simulink model "top_model"  (R2017b)
settings: Solver=FixedStepAuto  StartTime=0.0  StopTime=60000  FixedStep=.1  RelTol=1e-3  EnableMultiTasking=on
model workspace: external: MATLAB File C:\Users\Justin\Documents\00 MEng Project\PAN_ADCS\initialization\simulink_workspace_init.m (data not in the file)
undefined symbols (not defined in the file): h_init, hdmax, hmax, IAU, Imp_max, Imp_min, init, K_F, Kd, km, Kp, L_F, m_follower, match_tol, muE, ontime_max, ontime_min, q_init, s, Thrust_max, Thrust_min, wbn_init
libraries: aerolibtransform2 x9, hEemethod x8, aerolibconvert2 x6, aerolibgravity2 x5, sharedtransform x4, aerolibutil x4, aerolibcelestial x3, vrlib x2
(part 1 of 3)
settings Model: Creator=The MathWorks, Inc.  LastModifiedBy=Justin
settings DataIOCC: LimitDataPoints=on
settings OptimizationCC: LifeSpan=inf
settings DebuggingCC: AllowSymbolicDim=off  SFUnexpectedBacktrackingDiag=warning  SFNoUnconditionalDefaultTransitionDiag=warning  SFExecutionAtInitializationDiag=none
settings ModelReferenceCC: PropagateSignalLabelsOutOfModel=off
settings CodeAppCC: StateflowObjectComments=on
settings GRTTargetCC: TargetLangStandard=C89/C90 (ANSI)
settings ConfigComp: CovMetricSettings=dw  CovHtmlReporting=on  CovSaveCumulativeToWorkspaceVar=on  CovSaveSingleToWorkspaceVar=on  CovExternalEMLEnable=off

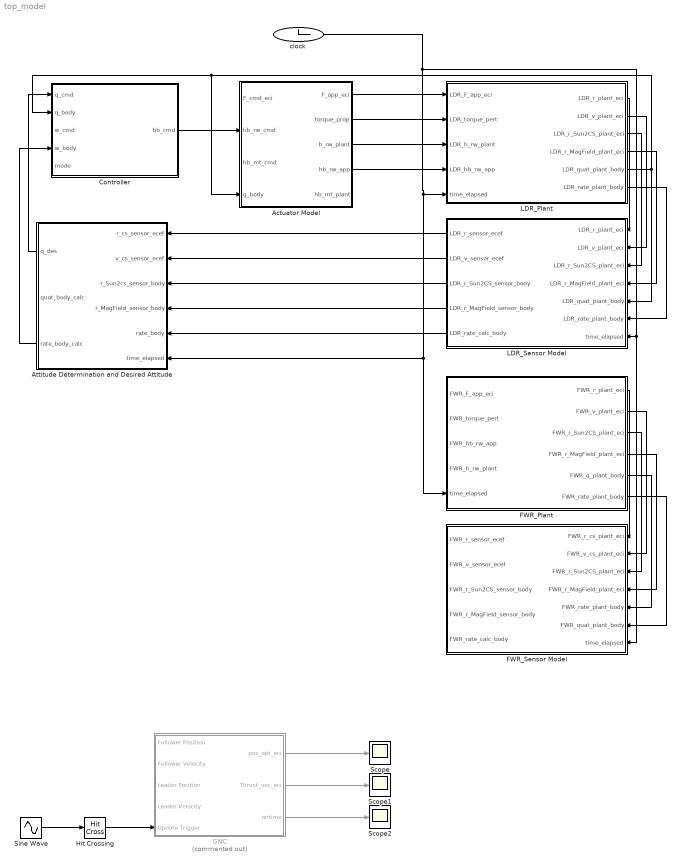
== system top_model ==
  Actuator Model : Subsystem
  Attitude Determination and Desired Attitude : Subsystem
  Controller : Subsystem
  FWR_Plant : Subsystem
  FWR_Sensor Model : Subsystem
  GNC : Subsystem  Commented=on
  Hit Crossing : HitCross  HitCrossingOffset=0.5  HitCrossingDirection=rising
  LDR_Plant : Subsystem
  LDR_Sensor Model : Subsystem
  Scope : Scope
  Scope1 : Scope
  Scope2 : Scope
  Sine Wave : Sin  Frequency=2*pi/5500  SampleTime=0
  clock : Clock
      settings: Decimation=100
  wires:
  clock/1 -> FWR_Sensor Model/7(time_elapsed), LDR_Sensor Model/7(time_elapsed), Attitude Determination and Desired Attitude/6(time_elapsed), FWR_Plant/5(time_elapsed), LDR_Plant/5(time_elapsed)
  LDR_Plant/1(LDR_r_plant_eci) -> LDR_Sensor Model/1(LDR_r_plant_eci)
  LDR_Plant/2(LDR_v_plant_eci) -> LDR_Sensor Model/2(LDR_v_plant_eci)
  LDR_Plant/3(LDR_r_Sun2CS_plant_eci) -> LDR_Sensor Model/3(LDR_r_Sun2CS_plant_eci)
  LDR_Plant/4(LDR_r_MagField_plant_eci) -> LDR_Sensor Model/4(LDR_r_MagField_plant_eci)
  LDR_Plant/6(LDR_rate_plant_body) -> LDR_Sensor Model/6(LDR_rate_plant_body)
  FWR_Plant/1(FWR_r_plant_eci) -> FWR_Sensor Model/1(FWR_r_cs_plant_eci)
  FWR_Plant/2(FWR_v_plant_eci) -> FWR_Sensor Model/2(FWR_v_cs_plant_eci)
  FWR_Plant/3(FWR_r_Sun2CS_plant_eci) -> FWR_Sensor Model/3(FWR_r_Sun2CS_plant_eci)
  FWR_Plant/4(FWR_r_MagField_plant_eci) -> FWR_Sensor Model/4(FWR_r_MagField_plant_eci)
  FWR_Plant/5(FWR_q_plant_body) -> FWR_Sensor Model/5(FWR_rate_plant_body)
  FWR_Plant/6(FWR_rate_plant_body) -> FWR_Sensor Model/6(FWR_quat_plant_body)
  Actuator Model/1(F_app_eci) -> LDR_Plant/1(LDR_F_app_eci)
  Actuator Model/2(torque_prop) -> LDR_Plant/2("LDR_torque_pert ")
  Actuator Model/3(h_rw_plant) -> LDR_Plant/3(LDR_h_rw_plant)
  Actuator Model/4(hb_rw_app) -> LDR_Plant/4(LDR_hb_rw_app)
  LDR_Sensor Model/1(LDR_r_sensor_ecef) -> Attitude Determination and Desired Attitude/1(r_cs_sensor_ecef)
  LDR_Sensor Model/2(LDR_v_sensor_ecef) -> Attitude Determination and Desired Attitude/2(v_cs_sensor_ecef)
  LDR_Sensor Model/3(LDR_r_Sun2CS_sensor_body) -> Attitude Determination and Desired Attitude/3(r_Sun2cs_sensor_body)
  LDR_Sensor Model/4(LDR_r_MagField_sensor_body) -> Attitude Determination and Desired Attitude/4(r_MagField_sensor_body)
  LDR_Sensor Model/5(LDR_rate_calc_body) -> Attitude Determination and Desired Attitude/5(rate_body)
  GNC/1(pos_opt_eci) -> Scope/1
  GNC/2(Thrust_vec_eci) -> Scope1/1
  GNC/3(ontime) -> Scope2/1
  Sine Wave/1 -> Hit Crossing/1
  Hit Crossing/1 -> GNC/5(Update Trigger)
  LDR_Plant/5(LDR_quat_plant_body) -> LDR_Sensor Model/5(LDR_quat_plant_body), Actuator Model/4(q_body), Controller/2(q_body)
  Attitude Determination and Desired Attitude/1(q_des) -> Controller/1(q_cmd)
  Attitude Determination and Desired Attitude/3(rate_body_calc) -> Controller/4(w_body)
  Controller/1(hb_cmd) -> Actuator Model/2(hb_rw_cmd)

== system top_model/Actuator Model ==
  F_cmd_eci : Inport
  hb_rw_cmd : Inport  Port=2
  hb_mt_cmd : Inport  Port=3
  q_body : Inport  Port=4
  Propulsion : Subsystem  Commented=on
  Rigid Body with Momentum Actuators and energy dissipation : Subsystem
  F_app_eci : Outport
  torque_prop : Outport  Port=2
  h_rw_plant : Outport  Port=3
  hb_rw_app : Outport  Port=4
  hb_mt_plant : Outport  Port=5
  wires:
  Rigid Body with Momentum Actuators and energy dissipation/1(LDR_h_RWA) -> h_rw_plant/1
  Rigid Body with Momentum Actuators and energy dissipation/2(LDR_hb_RWA) -> hb_rw_app/1
  hb_mt_cmd/1 -> hb_mt_plant/1
  F_cmd_eci/1 -> Propulsion/1(Force_cmd_eci)
  Propulsion/1(Force_applied) -> F_app_eci/1
  hb_rw_cmd/1 -> Rigid Body with Momentum Actuators and energy dissipation/1(hb)
  q_body/1 -> Rigid Body with Momentum Actuators and energy dissipation/2(q_body)

== system top_model/Attitude Determination and Desired Attitude ==
  r_cs_sensor_ecef : Inport
  v_cs_sensor_ecef : Inport  Port=2
  r_Sun2cs_sensor_body : Inport  Port=3
  r_MagField_sensor_body : Inport  Port=4
  rate_body : Inport  Port=5
  time_elapsed : Inport  Port=6
  Attitude Determination : Subsystem
  Demux1 : Demux
  Demux2 : Demux
  Direction Cosine Matrix to Quaternions : sharedtransform/Direction Cosine Matrix  to Quaternions  Commented=on
      settings: SourceProductName=Aerospace Blockset  SourceProductBaseCode=AE
  ECEF2ECI : Subsystem
  ECEF2ECI1 : Subsystem
  Position and Velocity to Desired Attitude in Quat : Subsystem
  Quaternions to Direction Cosine Matrix : sharedtransform/Quaternions to  Direction Cosine Matrix  Commented=on
      settings: SourceProductName=Aerospace Blockset  SourceProductBaseCode=AE
  Quaternions to Rotation Angles : sharedtransform/Quaternions to Rotation Angles  Commented=on  rotationOrder=ZYX
      settings: SourceProductBaseCode=AE
  Rotation Angles to Direction Cosine Matrix : sharedtransform/Rotation Angles to Direction Cosine Matrix  Commented=on  rotationOrder=ZYX
      settings: SourceProductBaseCode=AE
  q_calc : Scope  NumInputPorts=4
  q_ref : Scope  NumInputPorts=4
  q_des : Outport
  quat_body_calc : Outport  Port=2
  rate_body_calc : Outport  Port=3
  wires:
  rate_body/1 -> rate_body_calc/1
  time_elapsed/1 -> ECEF2ECI1/2(sec), ECEF2ECI/2(sec), Attitude Determination/1(time_elapsed)
  r_cs_sensor_ecef/1 -> ECEF2ECI/1(ecef)
  v_cs_sensor_ecef/1 -> ECEF2ECI1/1(ecef)
  ECEF2ECI/1(eci) -> Attitude Determination/2(r_cs_sensor_eci), Position and Velocity to Desired Attitude in Quat/1(r_cs_sensor_eci)
  ECEF2ECI1/1(eci) -> Position and Velocity to Desired Attitude in Quat/2(v_cs_sensor_eci)
  r_Sun2cs_sensor_body/1 -> Attitude Determination/3(r_Sun2cs_sensor_body)
  r_MagField_sensor_body/1 -> Attitude Determination/4(r_MagField_sensor_body)
  Attitude Determination/1(quat_body_calc) -> Demux1/1, quat_body_calc/1
  Demux1/2 -> q_calc/2
  Demux1/1 -> q_calc/1
  Demux1/3 -> q_calc/3
  Demux1/4 -> q_calc/4
  Position and Velocity to Desired Attitude in Quat/1(q_des) -> Demux2/1, q_des/1
  Demux2/2 -> q_ref/2
  Demux2/1 -> q_ref/1
  Demux2/3 -> q_ref/3
  Demux2/4 -> q_ref/4

== system top_model/Controller ==
  note: 0- Power ON / Restart
      | 1- Detumble
      | 2- Regulation Control
      | 3- Tracking Control
      | 4- Thermal Safe
      | 5- Power Max
      | 6- Large Angle Slew
  note: 0- Power ON/restart
      | 1- Safe hold
      | 2- Detumble
      | 3- Large angle slew
      | 4- Normal
      | 5- Eclipse
      | 6- Docking
  q_cmd : Inport
  q_body : Inport  Port=2
  w_cmd : Inport  Port=3
  w_body : Inport  Port=4
  mode : Inport  Port=5
  Free Rigid Body with Momentum Actuators2 : Subsystem  Commented=on
  If : If  IfExpression=u1 == 0  ElseIfExpressions=u1 == 1, u1 == 2, u1 == 3, u1 == 4, u1==5
  Mode Generator : Stateflow chart  Commented=on  TreatAsAtomicUnit=on
  Normal Mode Control System : Subsystem  TreatAsAtomicUnit=on
  TestNormalMode : Constant  Value=4
  hb_cmd : Outport
  wires:
  q_cmd/1 -> Mode Generator/2(q_cmd), Normal Mode Control System/1(q_cmd)
  q_body/1 -> Mode Generator/1(q_body), Normal Mode Control System/2(q_body)
  w_cmd/1 -> Normal Mode Control System/3(w_cmd)
  w_body/1 -> Mode Generator/3(w_body), Normal Mode Control System/4(w_body)
  TestNormalMode/1 -> If/1
  If/5 -> Normal Mode Control System/Action
  Normal Mode Control System/1(hb_cmd) -> hb_cmd/1

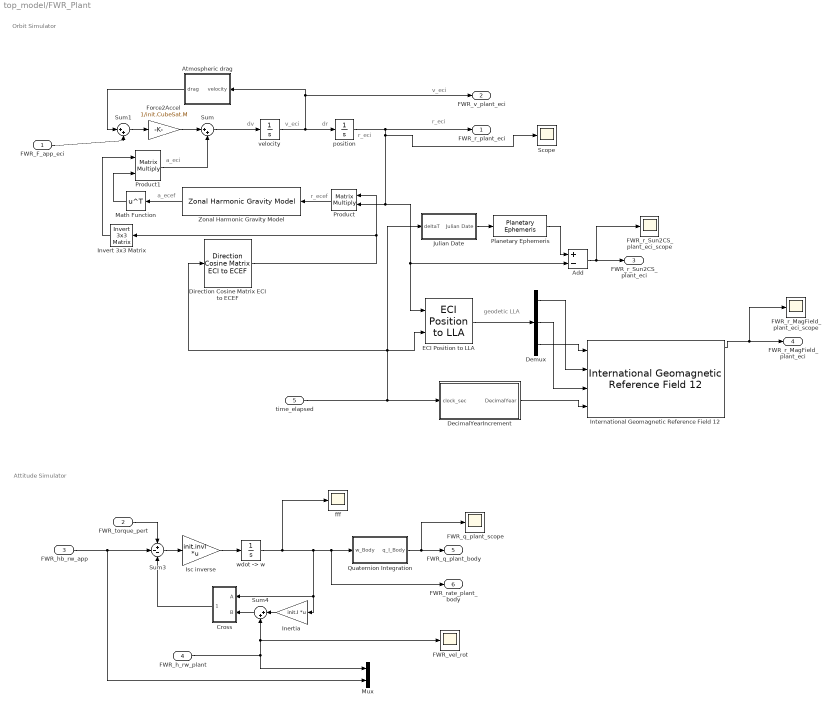
== system top_model/FWR_Plant ==
  note: Attitude Simulator
  note: dr
  note: r_eci
  note: r_eci
  note: dv
  note: v_eci
  note: Orbit Simulator
  note: r_ecef
  note: geodetic LLA
  note: a_eci
  note: v_eci
  note: a_ecef
  FWR_F_app_eci : Inport
  "FWR_torque_pert " : Inport  Port=2
  FWR_hb_rw_app : Inport  Port=3
  FWR_h_rw_plant : Inport  Port=4
  time_elapsed : Inport  Port=5
  Add : Sum  Inputs=+-
  Atmospheric drag : MATLAB Function  TreatAsAtomicUnit=on
  Cross : Subsystem
  DecimalYearIncrement : Subsystem
  Demux : Demux  Outputs=3
  Direction Cosine Matrix ECI to ECEF : aerolibtransform2/Direction Cosine Matrix ECI to ECEF  red=IAU-2000/2006  year=init.year  month=October  day=20  hour=init.hour  min=init.min  sec=init.sec  deltaT=Sec  errorflag=Error  extraparamflag=off
      settings: AttributesFormatString=%<red>  SourceProductName=Aerospace Blockset  SourceProductBaseCode=AE
  ECI Position to LLA : aerolibtransform2/ECI Position to LLA  red=IAU-2000/2006  year=init.year  month=October  day=20  hour=init.hour  min=init.min  sec=init.sec  deltaT=Sec  errorflag=Error  extraparamflag=off  eunits=Metric (MKS)  earthmodel=WGS84  flat=1/298.257223563  eqradius=6378137
      settings: AttributesFormatString=%<red>  SourceProductName=Aerospace Blockset  SourceProductBaseCode=AE
  FWR_q_plant_scope : Scope
  FWR_r_MagField_plant_eci_scope : Scope
  FWR_r_Sun2CS_plant_eci_scope : Scope
  "FWR_vel_rot " : Scope
  Force2Accel : Gain  Gain=1/init.CubeSat.M
  Inertia : Gain  Gain=init.I  Multiplication=Matrix(K*u)  SaturateOnIntegerOverflow=on  OutDataTypeStr=Inherit: Same as input  ParamDataTypeStr=Inherit: Same as input
  International Geomagnetic Reference Field 12 : aerolibgravity2/International Geomagnetic Reference Field 12  units=Metric (MKS)  time_in=on  month=January  day=1  year=2020  action=None  sv_out=off
      settings: SourceProductName=Aerospace Blockset  SourceProductBaseCode=AE
  Invert 3x3 Matrix : aerolibutil/Invert  3x3 Matrix
  Isc inverse : Gain  Gain=init.invI  Multiplication=Matrix(K*u)  SaturateOnIntegerOverflow=on  OutDataTypeStr=Inherit: Same as input  ParamDataTypeStr=Inherit: Same as input
  Julian Date : Subsystem
  Math Function : Math  Operator=transpose  SaturateOnIntegerOverflow=on
  Mux : Mux  Inputs=2
  Planetary Ephemeris : aerolibcelestial/Planetary Ephemeris  kmflag=km,km/s  epochflag=Julian date  de=DE430  nCenter=Earth  nTarget=Sun  errorflag=Error  velflag=off
      settings: SourceProductName=Aerospace Blockset  SourceProductBaseCode=AE
  Product : Product  Multiplication=Matrix(*)
  Product1 : Product  Multiplication=Matrix(*)
  Quaternion Integration : Subsystem
  Scope : Scope
  Sum : Sum  Inputs=|++
  Sum1 : Sum  Inputs=|++
  Sum3 : Sum  Inputs=+--  SaturateOnIntegerOverflow=on  InputSameDT=on  OutDataTypeStr=Inherit: Same as first input
  Sum4 : Sum  Inputs=|++
  Zonal Harmonic Gravity Model : aerolibgravity2/Zonal Harmonic Gravity Model  units=Metric (MKS)  degree=4  action=Warning  ptype=Earth  R=6378136.3  GM=398600441500000  jvalue=[1.0826269e-03 -2.5323000e-06 -1.6204000e-06]
      settings: SourceProductName=Aerospace Blockset  SourceProductBaseCode=AE
  fff : Scope
  position : Integrator  InitialCondition=init.FWR.P  ContinuousStateAttributes='position'
  velocity : Integrator  InitialCondition=init.FWR.V  ContinuousStateAttributes='velocity'
  "wdot -> w" : Integrator  InitialCondition=init.FWR.wbn
  FWR_r_plant_eci : Outport
  FWR_v_plant_eci : Outport  Port=2
  FWR_r_Sun2CS_plant_eci : Outport  Port=3
  FWR_r_MagField_plant_eci : Outport  Port=4
  FWR_q_plant_body : Outport  Port=5
  FWR_rate_plant_body : Outport  Port=6
  wires:
  Inertia/1 -> Sum4/1
  Quaternion Integration/1(q_I_Body) -> FWR_q_plant_scope/1, FWR_q_plant_body/1
  FWR_hb_rw_app/1 -> Sum3/2, Mux/2
  Sum3/1 -> Isc inverse/1
  "wdot -> w"/1 -> Quaternion Integration/1(w_Body), FWR_rate_plant_body/1, Cross/1(A), Inertia/1, fff/1
  Isc inverse/1 -> "wdot -> w"/1
  "FWR_torque_pert "/1 -> Sum3/1
  Sum4/1 -> Cross/2(B)
  Cross/1(AxB) -> Sum3/3
  FWR_h_rw_plant/1 -> Sum4/2, "FWR_vel_rot "/1, Mux/1
  time_elapsed/1 -> DecimalYearIncrement/1(clock_sec), ECI Position to LLA/2, Direction Cosine Matrix ECI to ECEF/1, Julian Date/1(deltaT)
  DecimalYearIncrement/1(DecimalYear) -> International Geomagnetic Reference Field 12/4
  International Geomagnetic Reference Field 12/1 -> FWR_r_MagField_plant_eci_scope/1, FWR_r_MagField_plant_eci/1
  Planetary Ephemeris/1 -> Add/1
  velocity/1 -> position/1, Atmospheric drag/1(velocity), FWR_v_plant_eci/1
  Force2Accel/1 -> Sum/1
  Demux/3 -> International Geomagnetic Reference Field 12/1
  Math Function/1 -> Product1/2
  Sum/1 -> velocity/1
  Product1/1 -> Sum/2
  Demux/1 -> International Geomagnetic Reference Field 12/2
  Atmospheric drag/1(drag) -> Sum1/1
  Product/1 -> Zonal Harmonic Gravity Model/1
  FWR_F_app_eci/1 -> Sum1/2
  Zonal Harmonic Gravity Model/1 -> Math Function/1
  position/1 -> Product/2, ECI Position to LLA/1, Add/2, Scope/1, FWR_r_plant_eci/1
  Demux/2 -> International Geomagnetic Reference Field 12/3
  Direction Cosine Matrix ECI to ECEF/1 -> Invert 3x3 Matrix/1, Product/1
  Invert 3x3 Matrix/1 -> Product1/1
  Julian Date/1(Julian Date) -> Planetary Ephemeris/1
  Sum1/1 -> Force2Accel/1
  ECI Position to LLA/1 -> Demux/1
  Add/1 -> FWR_r_Sun2CS_plant_eci_scope/1, FWR_r_Sun2CS_plant_eci/1

== system top_model/FWR_Sensor Model ==
  note: Gyroscope
  note: Magnetometer
  note: Sun Sensor
  note: GPS
  note: GPS
  FWR_r_cs_plant_eci : Inport
  FWR_v_cs_plant_eci : Inport  Port=2
  FWR_r_Sun2CS_plant_eci : Inport  Port=3
  FWR_r_MagField_plant_eci : Inport  Port=4
  FWR_rate_plant_body : Inport  Port=5
  FWR_quat_plant_body : Inport  Port=6
  time_elapsed : Inport  Port=7
  Direction Cosine Matrix ECI to ECEF : aerolibtransform2/Direction Cosine Matrix ECI to ECEF  red=IAU-2000/2006  year=init.year  month=October  day=20  hour=init.hour  min=init.min  sec=init.sec  deltaT=Sec  errorflag=Error  extraparamflag=off
      settings: AttributesFormatString=%<red>  SourceProductName=Aerospace Blockset  SourceProductBaseCode=AE
  Matrix Multiply : Product  Multiplication=Matrix(*)
  Matrix Multiply1 : Product  Multiplication=Matrix(*)
  FWR_r_sensor_ecef : Outport
  FWR_v_sensor_ecef : Outport  Port=2
  FWR_r_Sun2CS_sensor_body : Outport  Port=3
  FWR_r_MagField_sensor_body : Outport  Port=4
  FWR_rate_calc_body : Outport  Port=5
  wires:
  FWR_r_cs_plant_eci/1 -> Matrix Multiply/2
  FWR_r_Sun2CS_plant_eci/1 -> FWR_r_Sun2CS_sensor_body/1
  FWR_r_MagField_plant_eci/1 -> FWR_r_MagField_sensor_body/1
  FWR_rate_plant_body/1 -> FWR_rate_calc_body/1
  FWR_quat_plant_body/1 -> ?
  time_elapsed/1 -> Direction Cosine Matrix ECI to ECEF/1
  Direction Cosine Matrix ECI to ECEF/1 -> Matrix Multiply1/1, Matrix Multiply/1
  Matrix Multiply/1 -> FWR_r_sensor_ecef/1
  FWR_v_cs_plant_eci/1 -> Matrix Multiply1/2
  Matrix Multiply1/1 -> FWR_v_sensor_ecef/1

== system top_model/GNC ==
  Follower Position : Inport
  Follower Velocity : Inport  Port=2
  Leader Position : Inport  Port=3
  Leader Velocity : Inport  Port=4
  Update Trigger : Inport  Port=5
  Follower Maneuver : Subsystem
  Follower Orbital Elements : Subsystem
  Leader Orbital Elements : Subsystem
  Mux : Mux  Inputs=6
  Mux1 : Mux  Inputs=6
  Params : Subsystem
  Target Orbit : MATLAB Function  TreatAsAtomicUnit=on
  pos_opt_eci : Outport
  Thrust_vec_eci : Outport  Port=2
  ontime : Outport  Port=3
  wires:
  Follower Position/1 -> Follower Orbital Elements/1(r), Follower Maneuver/1(r_follower), Target Orbit/3(r_f)
  Follower Maneuver/2(pos_opt) -> pos_opt_eci/1
  [Imp_min] -> Follower Maneuver/7(Imp_min)
  Follower Maneuver/3(Thrust_vec) -> Thrust_vec_eci/1
  Leader Orbital Elements/4(Ω) -> Mux/4
  Mux/1 -> Target Orbit/5(els_t)
  Follower Orbital Elements/6(θ) -> Mux1/6
  Follower Orbital Elements/2(e) -> Mux1/2
  Follower Orbital Elements/3(i) -> Mux1/3
  Update Trigger/1 -> Follower Maneuver/8(Update Trigger)
  Leader Velocity/1 -> Leader Orbital Elements/2(v), Target Orbit/2(v_t)
  [Imp_max] -> Follower Maneuver/6(Imp_max)
  Target Orbit/1(x_tgt) -> Follower Maneuver/4(x_tgt)
  [muE] -> Follower Maneuver/3(mu), Target Orbit/7(muE)
  [match_tol] -> Target Orbit/9(match_tol)
  [m_f] -> Follower Maneuver/5(m_follower)
  Follower Velocity/1 -> Follower Orbital Elements/2(v), Follower Maneuver/2(v_follower), Target Orbit/4(v_f)
  Follower Orbital Elements/1(a) -> Mux1/1
  Follower Orbital Elements/4(Ω) -> Mux1/4
  Leader Orbital Elements/5(ω) -> Mux/5
  Follower Maneuver/4(ontime) -> ontime/1
  Mux1/1 -> Target Orbit/6(els_f)
  Leader Orbital Elements/3(i) -> Mux/3
  Follower Orbital Elements/5(ω) -> Mux1/5
  Leader Orbital Elements/6(θ) -> Mux/6
  Leader Position/1 -> Leader Orbital Elements/1(r), Target Orbit/1(r_t)
  Leader Orbital Elements/1(a) -> Mux/1
  Leader Orbital Elements/2(e) -> Mux/2
  [K_F] -> Target Orbit/8(K_F)

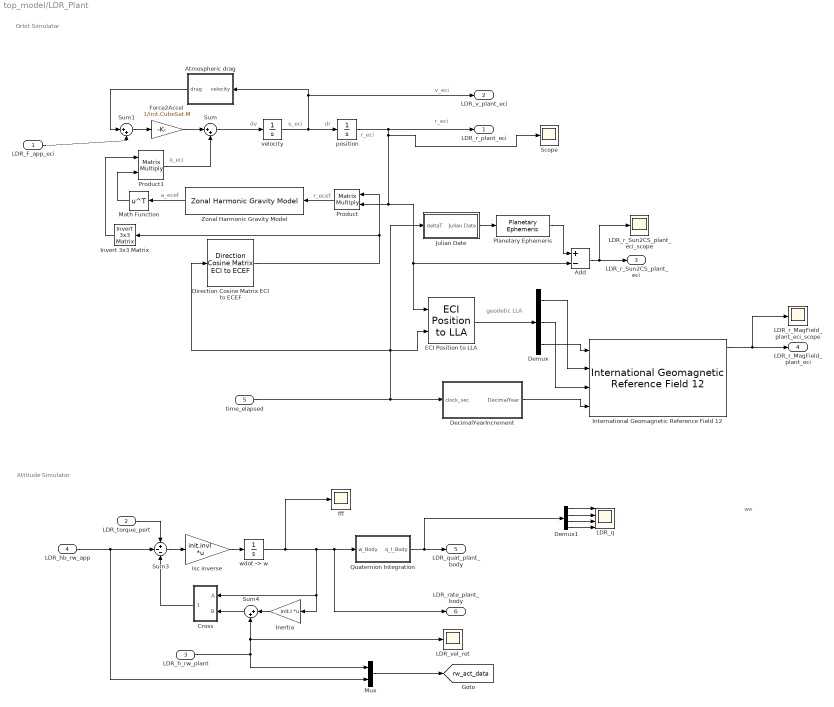
== system top_model/LDR_Plant ==
  note: we
  note: a_ecef
  note: v_eci
  note: a_eci
  note: geodetic LLA
  note: r_ecef
  note: Orbit Simulator
  note: v_eci
  note: dv
  note: r_eci
  note: r_eci
  note: dr
  note: Attitude Simulator
  LDR_F_app_eci : Inport
  "LDR_torque_pert " : Inport  Port=2
  LDR_h_rw_plant : Inport  Port=3
  LDR_hb_rw_app : Inport  Port=4
  time_elapsed : Inport  Port=5
  Add : Sum  Inputs=+-
  Atmospheric drag : MATLAB Function  TreatAsAtomicUnit=on
  Cross : Subsystem
  DecimalYearIncrement : Subsystem
  Demux : Demux  Outputs=3
  Demux1 : Demux
  Direction Cosine Matrix ECI to ECEF : aerolibtransform2/Direction Cosine Matrix ECI to ECEF  red=IAU-2000/2006  year=init.year  month=October  day=20  hour=init.hour  min=init.min  sec=init.sec  deltaT=Sec  errorflag=Error  extraparamflag=off
      settings: AttributesFormatString=%<red>  SourceProductName=Aerospace Blockset  SourceProductBaseCode=AE
  ECI Position to LLA : aerolibtransform2/ECI Position to LLA  red=IAU-2000/2006  year=init.year  month=October  day=20  hour=init.hour  min=init.min  sec=init.sec  deltaT=Sec  errorflag=Error  extraparamflag=off  eunits=Metric (MKS)  earthmodel=WGS84  flat=1/298.257223563  eqradius=6378137
      settings: AttributesFormatString=%<red>  SourceProductName=Aerospace Blockset  SourceProductBaseCode=AE
  Force2Accel : Gain  Gain=1/init.CubeSat.M
  Inertia : Gain  Gain=init.I  Multiplication=Matrix(K*u)  SaturateOnIntegerOverflow=on  OutDataTypeStr=Inherit: Same as input  ParamDataTypeStr=Inherit: Same as input
  International Geomagnetic Reference Field 12 : aerolibgravity2/International Geomagnetic Reference Field 12  units=Metric (MKS)  time_in=on  month=January  day=1  year=2020  action=None  sv_out=off
      settings: SourceProductName=Aerospace Blockset  SourceProductBaseCode=AE
  Invert 3x3 Matrix : aerolibutil/Invert  3x3 Matrix
  Isc inverse : Gain  Gain=init.invI  Multiplication=Matrix(K*u)  SaturateOnIntegerOverflow=on  OutDataTypeStr=Inherit: Same as input  ParamDataTypeStr=Inherit: Same as input
  Julian Date : Subsystem
  LDR_q : Scope  NumInputPorts=4
  LDR_r_MagField_plant_eci_scope : Scope
  LDR_r_Sun2CS_plant_eci_scope : Scope
  "LDR_vel_rot " : Scope
  Math Function : Math  Operator=transpose  SaturateOnIntegerOverflow=on
  Mux : Mux  Inputs=2
  Planetary Ephemeris : aerolibcelestial/Planetary Ephemeris  kmflag=km,km/s  epochflag=Julian date  de=DE430  nCenter=Earth  nTarget=Sun  errorflag=Error  velflag=off
      settings: SourceProductName=Aerospace Blockset  SourceProductBaseCode=AE
  Product : Product  Multiplication=Matrix(*)
  Product1 : Product  Multiplication=Matrix(*)
  Quaternion Integration : Subsystem
  Scope : Scope
  Sum : Sum  Inputs=|++
  Sum1 : Sum  Inputs=|++
  Sum3 : Sum  Inputs=+--  SaturateOnIntegerOverflow=on  InputSameDT=on  OutDataTypeStr=Inherit: Same as first input
  Sum4 : Sum  Inputs=|++
  Zonal Harmonic Gravity Model : aerolibgravity2/Zonal Harmonic Gravity Model  units=Metric (MKS)  degree=4  action=Warning  ptype=Earth  R=6378136.3  GM=398600441500000  jvalue=[1.0826269e-03 -2.5323000e-06 -1.6204000e-06]
      settings: SourceProductName=Aerospace Blockset  SourceProductBaseCode=AE
  fff : Scope
  position : Integrator  InitialCondition=init.LDR.P  ContinuousStateAttributes='position'
  velocity : Integrator  InitialCondition=init.LDR.V  ContinuousStateAttributes='velocity'
  "wdot -> w" : Integrator  InitialCondition=init.LDR.wbn
  LDR_r_plant_eci : Outport
  LDR_v_plant_eci : Outport  Port=2
  LDR_r_Sun2CS_plant_eci : Outport  Port=3
  LDR_r_MagField_plant_eci : Outport  Port=4
  LDR_quat_plant_body : Outport  Port=5
  LDR_rate_plant_body : Outport  Port=6
  tag scope: rw_act_data=global
  wires:
  Add/1 -> LDR_r_Sun2CS_plant_eci/1, LDR_r_Sun2CS_plant_eci_scope/1
  ECI Position to LLA/1 -> Demux/1
  Sum1/1 -> Force2Accel/1
  Julian Date/1(Julian Date) -> Planetary Ephemeris/1
  Invert 3x3 Matrix/1 -> Product1/1
  Direction Cosine Matrix ECI to ECEF/1 -> Product/1, Invert 3x3 Matrix/1
  Demux/2 -> International Geomagnetic Reference Field 12/3
  Zonal Harmonic Gravity Model/1 -> Math Function/1
  LDR_F_app_eci/1 -> Sum1/2
  Product/1 -> Zonal Harmonic Gravity Model/1
  Atmospheric drag/1(drag) -> Sum1/1
  Demux/1 -> International Geomagnetic Reference Field 12/2
  Product1/1 -> Sum/2
  Sum/1 -> velocity/1
  Math Function/1 -> Product1/2
  Demux/3 -> International Geomagnetic Reference Field 12/1
  Force2Accel/1 -> Sum/1
  velocity/1 -> LDR_v_plant_eci/1, Atmospheric drag/1(velocity), position/1
  Planetary Ephemeris/1 -> Add/1
  International Geomagnetic Reference Field 12/1 -> LDR_r_MagField_plant_eci/1, LDR_r_MagField_plant_eci_scope/1
  DecimalYearIncrement/1(DecimalYear) -> International Geomagnetic Reference Field 12/4
  time_elapsed/1 -> Julian Date/1(deltaT), Direction Cosine Matrix ECI to ECEF/1, ECI Position to LLA/2, DecimalYearIncrement/1(clock_sec)
  LDR_h_rw_plant/1 -> Mux/1, "LDR_vel_rot "/1, Sum4/2
  Cross/1(AxB) -> Sum3/3
  Sum4/1 -> Cross/2(B)
  "LDR_torque_pert "/1 -> Sum3/1
  Isc inverse/1 -> "wdot -> w"/1
  "wdot -> w"/1 -> fff/1, Inertia/1, Cross/1(A), LDR_rate_plant_body/1, Quaternion Integration/1(w_Body)
  Sum3/1 -> Isc inverse/1
  LDR_hb_rw_app/1 -> Mux/2, Sum3/2
  Mux/1 -> [rw_act_data]
  Inertia/1 -> Sum4/1
  Quaternion Integration/1(q_I_Body) -> Demux1/1, LDR_quat_plant_body/1
  Demux1/2 -> LDR_q/2
  Demux1/1 -> LDR_q/1
  Demux1/3 -> LDR_q/3
  Demux1/4 -> LDR_q/4
  position/1 -> LDR_r_plant_eci/1, Scope/1, Add/2, ECI Position to LLA/1, Product/2

== system top_model/LDR_Sensor Model ==
  note: Gyroscope
  note: Magnetometer
  note: Sun Sensor
  note: GPS
  note: GPS
  LDR_r_plant_eci : Inport
  LDR_v_plant_eci : Inport  Port=2
  LDR_r_Sun2CS_plant_eci : Inport  Port=3
  LDR_r_MagField_plant_eci : Inport  Port=4
  LDR_quat_plant_body : Inport  Port=5
  LDR_rate_plant_body : Inport  Port=6
  time_elapsed : Inport  Port=7
  Direction Cosine Matrix ECI to ECEF : aerolibtransform2/Direction Cosine Matrix ECI to ECEF  red=IAU-2000/2006  year=init.year  month=October  day=20  hour=init.hour  min=init.min  sec=init.sec  deltaT=Sec  errorflag=Error  extraparamflag=off
      settings: AttributesFormatString=%<red>  SourceProductName=Aerospace Blockset  SourceProductBaseCode=AE
  Matrix Multiply{,1..3} (4 alike) : Product  Multiplication=Matrix(*)
  quat to DCM : Subsystem  mask(Direction Cosine Matrix){}
      mask help: Determines the 3x3 Direction Cosine Matrix (DCM) from a 4x1 quaternion orientation vector. The outputted DCM transforms vectors from inertial axes to body axes. This version corrects the fucked-up MATLAB one.
      mask Help:
      | <p>This block determines the 3x3 Direction Cosine Matrix (DCM) from a 4x1 quaternion orientation vector. The outputted DCM transforms vectors from inertial axes to body axes.  This version corrects the fucked-up MATLAB one</p>
      | 
      | <p>The block input and output contain more than one signal as described below.</p>
      | 
      | <p><H4>Block Vector Input - Quaternion</H4>
      | <ul>
      | <li>q0</li>
      | <li>q1</li>
      | <li>q2</li>
      | <li>q3</li>
      | </ul>
      | </p>
      | 
      | <p><H4>Block Matrix Output - Direction Cosine Matrix  </H4>
      |     <ul>
      |    </ul>
      |    </p>
      mask Display: disp('q to Q')
  LDR_r_sensor_ecef : Outport
  LDR_v_sensor_ecef : Outport  Port=2
  LDR_r_Sun2CS_sensor_body : Outport  Port=3
  LDR_r_MagField_sensor_body : Outport  Port=4
  LDR_rate_calc_body : Outport  Port=5
  wires:
  LDR_r_plant_eci/1 -> Matrix Multiply/2
  LDR_rate_plant_body/1 -> LDR_rate_calc_body/1
  LDR_quat_plant_body/1 -> quat to DCM/1(e0 e1 e2 e3)
  time_elapsed/1 -> Direction Cosine Matrix ECI to ECEF/1
  Direction Cosine Matrix ECI to ECEF/1 -> Matrix Multiply1/1, Matrix Multiply/1
  Matrix Multiply/1 -> LDR_r_sensor_ecef/1
  LDR_v_plant_eci/1 -> Matrix Multiply1/2
  Matrix Multiply1/1 -> LDR_v_sensor_ecef/1
  LDR_r_Sun2CS_plant_eci/1 -> Matrix Multiply3/2
  LDR_r_MagField_plant_eci/1 -> Matrix Multiply2/2
  Matrix Multiply3/1 -> LDR_r_Sun2CS_sensor_body/1
  Matrix Multiply2/1 -> LDR_r_MagField_sensor_body/1
  quat to DCM/1(DCM) -> Matrix Multiply3/1, Matrix Multiply2/1

== system top_model/Actuator Model/Propulsion ==
  Force_cmd_eci : Inport
  MATLAB Function : MATLAB Function  TreatAsAtomicUnit=on
  Force_applied : Outport
  wires:
  Force_cmd_eci/1 -> MATLAB Function/1(Target)

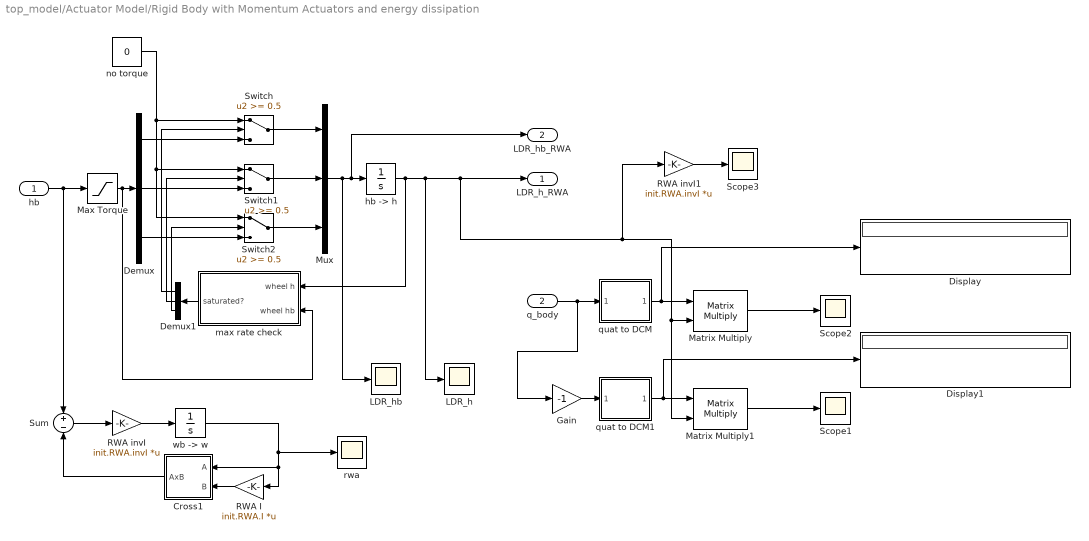
== system top_model/Actuator Model/Rigid Body with Momentum Actuators and energy dissipation ==
  hb : Inport
  q_body : Inport  Port=2
  Cross1 : Subsystem
  Demux : Demux  Outputs=3
  Demux1 : Demux  Outputs=3
  Display : Display
  Display1 : Display
  Gain : Gain  Gain=-1
  LDR_h : Scope
  LDR_hb : Scope
  Matrix Multiply : Product  Multiplication=Matrix(*)
  Matrix Multiply1 : Product  Multiplication=Matrix(*)
  Max Torque : Saturate  UpperLimit=init.hdmax  LowerLimit=-init.hdmax
  Mux : Mux  Inputs=3
  RWA I : Gain  Gain=init.RWA.I  Multiplication=Matrix(K*u)
  RWA invI : Gain  Gain=init.RWA.invI  Multiplication=Matrix(K*u)
  RWA invI1 : Gain  Gain=init.RWA.invI  Multiplication=Matrix(K*u)
  Scope1 : Scope
  Scope2 : Scope
  Scope3 : Scope
  Sum : Sum  Inputs=+|-
  Switch : Switch  Threshold=0.5  SaturateOnIntegerOverflow=on  InputSameDT=on
  Switch1 : Switch  Threshold=0.5  SaturateOnIntegerOverflow=on  InputSameDT=on
  Switch2 : Switch  Threshold=0.5  SaturateOnIntegerOverflow=on  InputSameDT=on
  "hb -> h" : Integrator  InitialCondition=init.LDR.h
  max rate check : Subsystem
  no torque : Constant  Value=0
  quat to DCM : Subsystem  mask(Direction Cosine Matrix){}
      mask help: Determines the 3x3 Direction Cosine Matrix (DCM) from a 4x1 quaternion orientation vector. The outputted DCM transforms vectors from inertial axes to body axes. This version corrects the fucked-up MATLAB one.
      mask Help:
      | <p>This block determines the 3x3 Direction Cosine Matrix (DCM) from a 4x1 quaternion orientation vector. The outputted DCM transforms vectors from inertial axes to body axes.  This version corrects the fucked-up MATLAB one</p>
      | 
      | <p>The block input and output contain more than one signal as described below.</p>
      | 
      | <p><H4>Block Vector Input - Quaternion</H4>
      | <ul>
      | <li>q0</li>
      | <li>q1</li>
      | <li>q2</li>
      | <li>q3</li>
      | </ul>
      | </p>
      | 
      | <p><H4>Block Matrix Output - Direction Cosine Matrix  </H4>
      |     <ul>
      |    </ul>
      |    </p>
      mask Display: disp('q to Q')
  quat to DCM1 : Subsystem  mask(Direction Cosine Matrix){}
      mask help: Determines the 3x3 Direction Cosine Matrix (DCM) from a 4x1 quaternion orientation vector. The outputted DCM transforms vectors from inertial axes to body axes. This version corrects the fucked-up MATLAB one.
      mask Help:
      | <p>This block determines the 3x3 Direction Cosine Matrix (DCM) from a 4x1 quaternion orientation vector. The outputted DCM transforms vectors from inertial axes to body axes.  This version corrects the fucked-up MATLAB one</p>
      | 
      | <p>The block input and output contain more than one signal as described below.</p>
      | 
      | <p><H4>Block Vector Input - Quaternion</H4>
      | <ul>
      | <li>q0</li>
      | <li>q1</li>
      | <li>q2</li>
      | <li>q3</li>
      | </ul>
      | </p>
      | 
      | <p><H4>Block Matrix Output - Direction Cosine Matrix  </H4>
      |     <ul>
      |    </ul>
      |    </p>
      mask Display: disp('q to Q')
  rwa : Scope
  "wb -> w" : Integrator  InitialCondition=[0;0;0]
  LDR_h_RWA : Outport
  LDR_hb_RWA : Outport  Port=2
  wires:
  hb/1 -> Max Torque/1, Sum/1
  Mux/1 -> LDR_hb_RWA/1, "hb -> h"/1, LDR_hb/1
  Max Torque/1 -> Demux/1, max rate check/2(wheel hb)
  max rate check/1(saturated?) -> Demux1/1
  Demux1/1 -> Switch/2
  Demux1/2 -> Switch1/2
  Demux1/3 -> Switch2/2
  no torque/1 -> Switch/1, Switch1/1, Switch2/1
  Demux/1 -> Switch/3
  Demux/2 -> Switch1/3
  Demux/3 -> Switch2/3
  Switch/1 -> Mux/1
  Switch1/1 -> Mux/2
  Switch2/1 -> Mux/3
  q_body/1 -> Gain/1, quat to DCM/1(e0 e1 e2 e3)
  quat to DCM/1(DCM) -> Display/1, Matrix Multiply/1
  Matrix Multiply/1 -> Scope2/1
  Matrix Multiply1/1 -> Scope1/1
  quat to DCM1/1(DCM) -> Display1/1, Matrix Multiply1/1
  "hb -> h"/1 -> max rate check/1(wheel h), RWA invI1/1, Matrix Multiply1/2, Matrix Multiply/2, LDR_h_RWA/1, LDR_h/1
  Gain/1 -> quat to DCM1/1(e0 e1 e2 e3)
  RWA I/1 -> Cross1/2(B)
  "wb -> w"/1 -> rwa/1, Cross1/1(A), RWA I/1
  Cross1/1(AxB) -> Sum/2
  Sum/1 -> RWA invI/1
  RWA invI/1 -> "wb -> w"/1
  RWA invI1/1 -> Scope3/1

== system top_model/Attitude Determination and Desired Attitude/Attitude Determination ==
  time_elapsed : Inport
  r_cs_sensor_eci : Inport  Port=2
  r_Sun2cs_sensor_body : Inport  Port=3
  r_MagField_sensor_body : Inport  Port=4
  Generate reference vectors from Ephemeris and Magnetic Field Model : Subsystem
  Subsystem : Subsystem
  quat_body_calc : Outport
  wires:
  r_cs_sensor_eci/1 -> Generate reference vectors from Ephemeris and Magnetic Field Model/2(r_cs_sensor_eci)
  time_elapsed/1 -> Generate reference vectors from Ephemeris and Magnetic Field Model/1(time_elapsed)
  r_Sun2cs_sensor_body/1 -> Subsystem/3(r_Sun2cs_sensor_body)
  r_MagField_sensor_body/1 -> Subsystem/4(r_MagField_sensor_body)
  Generate reference vectors from Ephemeris and Magnetic Field Model/1(r_Sun2cs_ref_eci) -> Subsystem/1(r_Sun2cs_ref_eci)
  Generate reference vectors from Ephemeris and Magnetic Field Model/2(r_MagField_ref_eci) -> Subsystem/2(r_MagField_ref_eci)
  Subsystem/1(quat_body_calc) -> quat_body_calc/1

== system top_model/Attitude Determination and Desired Attitude/ECEF2ECI ==
  ecef : Inport
  sec : Inport  Port=2
  Direction Cosine Matrix ECI to ECEF : aerolibtransform2/Direction Cosine Matrix ECI to ECEF  red=IAU-2000/2006  year=init.year  month=October  day=20  hour=init.hour  min=init.min  sec=init.sec  deltaT=Sec  errorflag=Error  extraparamflag=off
      settings: AttributesFormatString=%<red>  SourceProductName=Aerospace Blockset  SourceProductBaseCode=AE
  Invert 3x3 Matrix : aerolibutil/Invert  3x3 Matrix
  Product1 : Product  Multiplication=Matrix(*)
  eci : Outport
  wires:
  Direction Cosine Matrix ECI to ECEF/1 -> Invert 3x3 Matrix/1
  Product1/1 -> eci/1
  sec/1 -> Direction Cosine Matrix ECI to ECEF/1
  Invert 3x3 Matrix/1 -> Product1/1
  ecef/1 -> Product1/2

== system top_model/Attitude Determination and Desired Attitude/ECEF2ECI1 ==
  ecef : Inport
  sec : Inport  Port=2
  Direction Cosine Matrix ECI to ECEF : aerolibtransform2/Direction Cosine Matrix ECI to ECEF  red=IAU-2000/2006  year=init.year  month=October  day=20  hour=init.hour  min=init.min  sec=init.sec  deltaT=Sec  errorflag=Error  extraparamflag=off
      settings: AttributesFormatString=%<red>  SourceProductName=Aerospace Blockset  SourceProductBaseCode=AE
  Invert 3x3 Matrix : aerolibutil/Invert  3x3 Matrix
  Product1 : Product  Multiplication=Matrix(*)
  eci : Outport
  wires:
  Direction Cosine Matrix ECI to ECEF/1 -> Invert 3x3 Matrix/1
  Product1/1 -> eci/1
  sec/1 -> Direction Cosine Matrix ECI to ECEF/1
  ecef/1 -> Product1/2
  Invert 3x3 Matrix/1 -> Product1/1

== system top_model/Attitude Determination and Desired Attitude/Position and Velocity to Desired Attitude in Quat ==
  r_cs_sensor_eci : Inport
  v_cs_sensor_eci : Inport  Port=2
  CreateDCM_be : Subsystem
  Display : Display
  Display1 : Display
  MATLAB Function : MATLAB Function  TreatAsAtomicUnit=on
  Memory : Memory
  Product : Product  Multiplication=Matrix(*)
  To Workspace1 : ToWorkspace  VariableName=tr  SampleTime=-1
  To Workspace2 : ToWorkspace  VariableName=q  SampleTime=-1
  To Workspace3 : ToWorkspace  VariableName=flag  SampleTime=-1
  dcm2quat : MATLAB Function  TreatAsAtomicUnit=on
  quat to DCM : Subsystem  mask(Direction Cosine Matrix){}
      mask help: Determines the 3x3 Direction Cosine Matrix (DCM) from a 4x1 quaternion orientation vector. The outputted DCM transforms vectors from inertial axes to body axes. This version corrects the fucked-up MATLAB one.
      mask Help:
      | <p>This block determines the 3x3 Direction Cosine Matrix (DCM) from a 4x1 quaternion orientation vector. The outputted DCM transforms vectors from inertial axes to body axes.  This version corrects the fucked-up MATLAB one</p>
      | 
      | <p>The block input and output contain more than one signal as described below.</p>
      | 
      | <p><H4>Block Vector Input - Quaternion</H4>
      | <ul>
      | <li>q0</li>
      | <li>q1</li>
      | <li>q2</li>
      | <li>q3</li>
      | </ul>
      | </p>
      | 
      | <p><H4>Block Matrix Output - Direction Cosine Matrix  </H4>
      |     <ul>
      |    </ul>
      |    </p>
      mask Display: disp('q to Q')
  q_des : Outport
  wires:
  r_cs_sensor_eci/1 -> CreateDCM_be/1(Position)
  v_cs_sensor_eci/1 -> CreateDCM_be/2(Velocity)
  dcm2quat/1(q) -> Memory/1, To Workspace2/1
  CreateDCM_be/1(DCM_be) -> dcm2quat/1(DCM_be), MATLAB Function/1(DCM_be), Product/2, Display/1
  dcm2quat/2(tr) -> To Workspace1/1
  dcm2quat/3(flag) -> To Workspace3/1
  Memory/1 -> dcm2quat/2(q_prev)
  Product/1 -> Display1/1
  quat to DCM/1(DCM) -> Product/1
  MATLAB Function/1(q) -> q_des/1

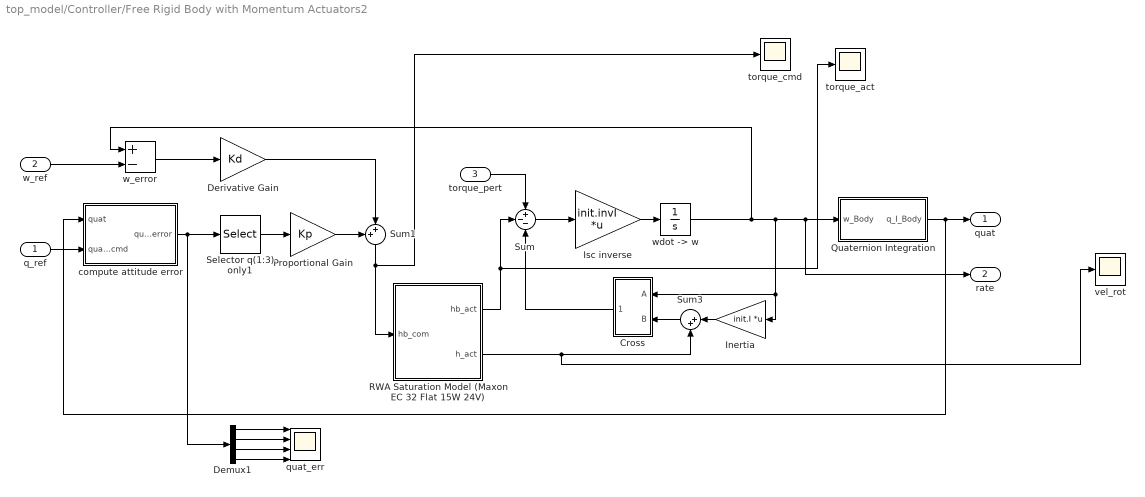
== system top_model/Controller/Free Rigid Body with Momentum Actuators2 ==
  q_ref : Inport
  w_ref : Inport  Port=2
  "torque_pert " : Inport  Port=3
  Cross : Subsystem
  Demux1 : Demux
  Derivative Gain : Gain  Gain=Kd  SaturateOnIntegerOverflow=on  OutDataTypeStr=Inherit: Same as input  ParamDataTypeStr=Inherit: Same as input
  Inertia : Gain  Gain=init.I  Multiplication=Matrix(K*u)  SaturateOnIntegerOverflow=on  OutDataTypeStr=Inherit: Same as input  ParamDataTypeStr=Inherit: Same as input
  Isc inverse : Gain  Gain=init.invI  Multiplication=Matrix(K*u)  SaturateOnIntegerOverflow=on  OutDataTypeStr=Inherit: Same as input  ParamDataTypeStr=Inherit: Same as input
  Proportional Gain : Gain  Gain=Kp  SaturateOnIntegerOverflow=on  OutDataTypeStr=Inherit: Same as input  ParamDataTypeStr=Inherit: Same as input
  Quaternion Integration : Subsystem
  RWA Saturation Model (Maxon EC 32 Flat 15W 24V) : Subsystem
  Selector q(1:3) only1 : Selector  InputPortWidth=4  IndexOptions=Index vector (dialog)  Indices=[1 2 3]  OutputSizes=1
  Sum : Sum  Inputs=+--  SaturateOnIntegerOverflow=on  InputSameDT=on  OutDataTypeStr=Inherit: Same as first input
  Sum1 : Sum  Inputs=++|
  Sum3 : Sum  Inputs=|++
  compute attitude error : Subsystem
  quat_err : Scope  NumInputPorts=4
  torque_act : Scope
  torque_cmd : Scope
  "vel_rot " : Scope
  w_error : Sum  Inputs=+-
  "wdot -> w" : Integrator  InitialCondition=wbn_init
  quat : Outport
  rate : Outport  Port=2
  wires:
  Sum/1 -> Isc inverse/1
  Isc inverse/1 -> "wdot -> w"/1
  Cross/1(AxB) -> Sum/3
  Quaternion Integration/1(q_I_Body) -> compute attitude error/1(quat), quat/1
  q_ref/1 -> compute attitude error/2(quat_cmd)
  Selector q(1:3) only1/1 -> Proportional Gain/1
  w_error/1 -> Derivative Gain/1
  w_ref/1 -> w_error/2
  "wdot -> w"/1 -> w_error/1, Inertia/1, Cross/1(A), Quaternion Integration/1(w_Body), rate/1
  Demux1/4 -> quat_err/4
  Demux1/1 -> quat_err/1
  compute attitude error/1(quat error) -> Demux1/1, Selector q(1:3) only1/1
  Demux1/2 -> quat_err/2
  Demux1/3 -> quat_err/3
  "torque_pert "/1 -> Sum/1
  Derivative Gain/1 -> Sum1/2
  Proportional Gain/1 -> Sum1/1
  Sum3/1 -> Cross/2(B)
  Inertia/1 -> Sum3/1
  RWA Saturation Model (Maxon EC 32 Flat 15W 24V)/2(h_act) -> "vel_rot "/1, Sum3/2
  Sum1/1 -> torque_cmd/1, RWA Saturation Model (Maxon EC 32 Flat 15W 24V)/1(hb_com)
  RWA Saturation Model (Maxon EC 32 Flat 15W 24V)/1(hb_act) -> Sum/2, torque_act/1

== system top_model/Controller/Normal Mode Control System ==
  q_cmd : Inport
  q_body : Inport  Port=2
  w_cmd : Inport  Port=3
  w_body : Inport  Port=4
  Action Port : ActionPort  PropagateVarSize=During execution  ActionType=elseif
  Constant : Constant  Value=[0;0;0]
  Demux1 : Demux
  Derivative Gain : Gain  Gain=Kd  SaturateOnIntegerOverflow=on  OutDataTypeStr=Inherit: Same as input  ParamDataTypeStr=Inherit: Same as input
  Proportional Gain : Gain  Gain=Kp  SaturateOnIntegerOverflow=on  OutDataTypeStr=Inherit: Same as input  ParamDataTypeStr=Inherit: Same as input
  Selector q(1:3) only1 : Selector  InputPortWidth=4  IndexOptions=Index vector (dialog)  Indices=[1 2 3]  OutputSizes=1
  Sum1 : Sum  Inputs=++|
  compute attitude error : Subsystem
  quat_err : Scope  NumInputPorts=4
  w_error : Sum  Inputs=+-
  hb_cmd : Outport
  wires:
  Proportional Gain/1 -> Sum1/1
  Derivative Gain/1 -> Sum1/2
  Demux1/2 -> quat_err/2
  w_error/1 -> Derivative Gain/1
  Demux1/3 -> quat_err/3
  Demux1/1 -> quat_err/1
  compute attitude error/1(quat error) -> Demux1/1, Selector q(1:3) only1/1
  w_body/1 -> w_error/1
  q_body/1 -> compute attitude error/1(quat)
  Demux1/4 -> quat_err/4
  q_cmd/1 -> compute attitude error/2(quat_cmd)
  Selector q(1:3) only1/1 -> Proportional Gain/1
  Sum1/1 -> hb_cmd/1
  Constant/1 -> w_error/2

== system top_model/FWR_Plant/Cross ==
  A : Inport
  B : Inport  Port=2
  Mux4 : Mux  Inputs=3
  Product{,1..5} (6 alike) : Product  SaturateOnIntegerOverflow=on  InputSameDT=on  OutDataTypeStr=Inherit: Same as first input
  Sum : Sum  Inputs=+-  SaturateOnIntegerOverflow=on  InputSameDT=on  OutDataTypeStr=Inherit: Same as first input
  Sum1 : Sum  Inputs=+-  SaturateOnIntegerOverflow=on  InputSameDT=on  OutDataTypeStr=Inherit: Same as first input
  Sum2 : Sum  Inputs=+-  SaturateOnIntegerOverflow=on  InputSameDT=on  OutDataTypeStr=Inherit: Same as first input
  demux2 : Demux  Outputs=3
  demux3 : Demux  Outputs=3
  AxB : Outport  InitialOutput=0
  wires:
  A/1 -> demux2/1
  B/1 -> demux3/1
  demux2/3 -> Product1/1, Product2/1
  demux3/3 -> Product/2, Product3/2
  demux2/1 -> Product3/1, Product4/1
  demux3/2 -> Product1/2, Product4/2
  demux2/2 -> Product/1, Product5/1
  demux3/1 -> Product2/2, Product5/2
  Product/1 -> Sum/1
  Product1/1 -> Sum/2
  Product2/1 -> Sum1/1
  Product3/1 -> Sum1/2
  Product4/1 -> Sum2/1
  Product5/1 -> Sum2/2
  Sum/1 -> Mux4/1
  Sum1/1 -> Mux4/2
  Sum2/1 -> Mux4/3
  Mux4/1 -> AxB/1

== system top_model/FWR_Plant/DecimalYearIncrement ==
  note: day
  clock_sec : Inport
  Add : Sum
  Constant : Constant  Value=init.year
  Constant1 : Constant  Value=init.month
  Constant2 : Constant  Value=init.day
  Constant3 : Constant  Value=init.hour
  Constant4 : Constant  Value=init.min
  Constant5 : Constant  Value=init.min
  Divide : Product  Inputs=*/
  MATLAB Function : MATLAB Function  TreatAsAtomicUnit=on
  Product2 : Product  Inputs=*/
  day2decimalYear : Constant  Value=365
  sec2day : Constant  Value=86400
  DecimalYear : Outport
  wires:
  Constant2/1 -> MATLAB Function/3(day)
  clock_sec/1 -> Product2/1
  Constant5/1 -> MATLAB Function/6(second)
  Constant4/1 -> MATLAB Function/5(minute)
  Constant/1 -> MATLAB Function/1(year)
  Constant1/1 -> MATLAB Function/2(month)
  MATLAB Function/1(DecimalYear) -> Add/2
  Divide/1 -> Add/1
  day2decimalYear/1 -> Divide/2
  Constant3/1 -> MATLAB Function/4(hour)
  Add/1 -> DecimalYear/1
  sec2day/1 -> Product2/2
  Product2/1 -> Divide/1

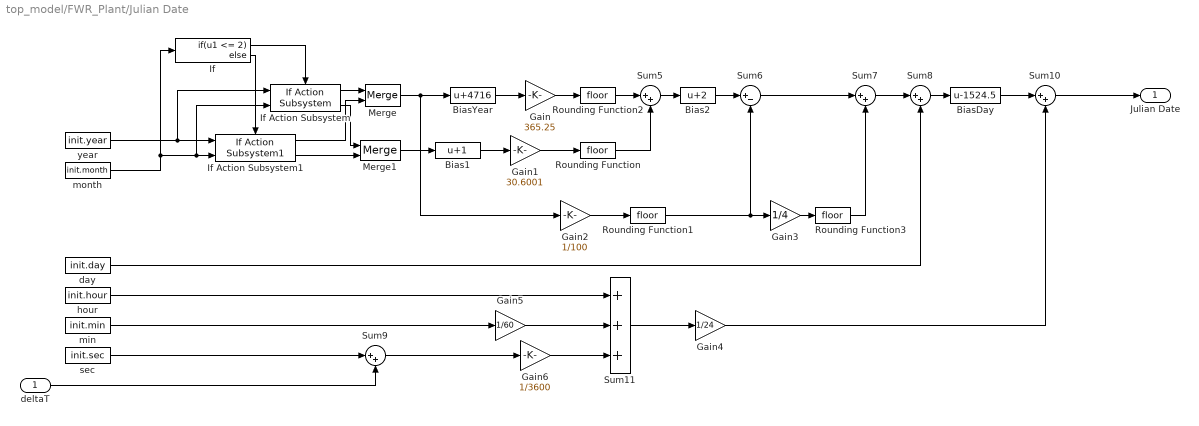
== system top_model/FWR_Plant/Julian Date ==
  deltaT : Inport  OutMin=0  PortDimensions=1
  Bias1 : Bias  Bias=1
  Bias2 : Bias  Bias=2
  BiasDay : Bias  Bias=-1524.5
  BiasYear : Bias  Bias=4716
  Gain : Gain  Gain=365.25
  Gain1 : Gain  Gain=30.6001
  Gain2 : Gain  Gain=1/100
  Gain3 : Gain  Gain=1/4
  Gain4 : Gain  Gain=1/24
  Gain5 : Gain  Gain=1/60
  Gain6 : Gain  Gain=1/3600
  If : If  IfExpression=u1 <= 2
  If Action Subsystem : aerolibconvert2/Julian Date Conversion/If Action Subsystem
      settings: SourceProductName=Aerospace Blockset  SourceProductBaseCode=AE
  If Action Subsystem1 : aerolibconvert2/Julian Date Conversion/If Action Subsystem1
      settings: SourceProductName=Aerospace Blockset  SourceProductBaseCode=AE
  Merge : Merge
  Merge1 : Merge
  Rounding Function{,1..3} (4 alike) : Rounding
  Sum{5,7..10} (5 alike) : Sum  Inputs=|++
  Sum11 : Sum  Inputs=+++
  Sum6 : Sum  Inputs=|+-
  day : Constant  Value=init.day
  hour : Constant  Value=init.hour
  min : Constant  Value=init.min
  month : Constant  Value=init.month
  sec : Constant  Value=init.sec
  year : Constant  Value=init.year
  Julian Date : Outport
  wires:
  Gain4/1 -> Sum10/2
  month/1 -> If/1, If Action Subsystem1/2, If Action Subsystem/2
  Rounding Function/1 -> Sum5/2
  Rounding Function2/1 -> Sum5/1
  Sum8/1 -> BiasDay/1
  Bias2/1 -> Sum6/1
  Rounding Function1/1 -> Sum6/2, Gain3/1
  Gain1/1 -> Rounding Function/1
  BiasDay/1 -> Sum10/1
  Sum5/1 -> Bias2/1
  If Action Subsystem1/2 -> Merge1/2
  sec/1 -> Sum9/1
  Bias1/1 -> Gain1/1
  day/1 -> Sum8/2
  Sum10/1 -> Julian Date/1
  Sum7/1 -> Sum8/1
  If Action Subsystem1/1 -> Merge/2
  hour/1 -> Sum11/1
  Gain3/1 -> Rounding Function3/1
  Sum11/1 -> Gain4/1
  Gain6/1 -> Sum11/3
  min/1 -> Gain5/1
  BiasYear/1 -> Gain/1
  Gain5/1 -> Sum11/2
  Sum6/1 -> Sum7/1
  Sum9/1 -> Gain6/1
  Merge/1 -> BiasYear/1, Gain2/1
  Gain2/1 -> Rounding Function1/1
  Gain/1 -> Rounding Function2/1
  Merge1/1 -> Bias1/1
  deltaT/1 -> Sum9/2
  Rounding Function3/1 -> Sum7/2
  If Action Subsystem/2 -> Merge1/1
  If/1 -> If Action Subsystem/Action
  year/1 -> If Action Subsystem1/1, If Action Subsystem/1
  If/2 -> If Action Subsystem1/Action
  If Action Subsystem/1 -> Merge/1

== system top_model/FWR_Plant/Quaternion Integration ==
  w_Body : Inport
  Constant : Constant  Value=[0.707, 0, 0,-0.707]
  Integrator1 : Integrator  InitialConditionSource=external  InitialCondition=q_init  ContinuousStateAttributes='quaternion_plant'
  q_normalize : Subsystem
  qderiv : Subsystem
  q_I_Body : Outport
  wires:
  Constant/1 -> Integrator1/2
  w_Body/1 -> qderiv/1(w)
  q_normalize/1(q_out) -> qderiv/2(q), q_I_Body/1
  Integrator1/1 -> q_normalize/1(q_in)
  qderiv/1(qd) -> Integrator1/1

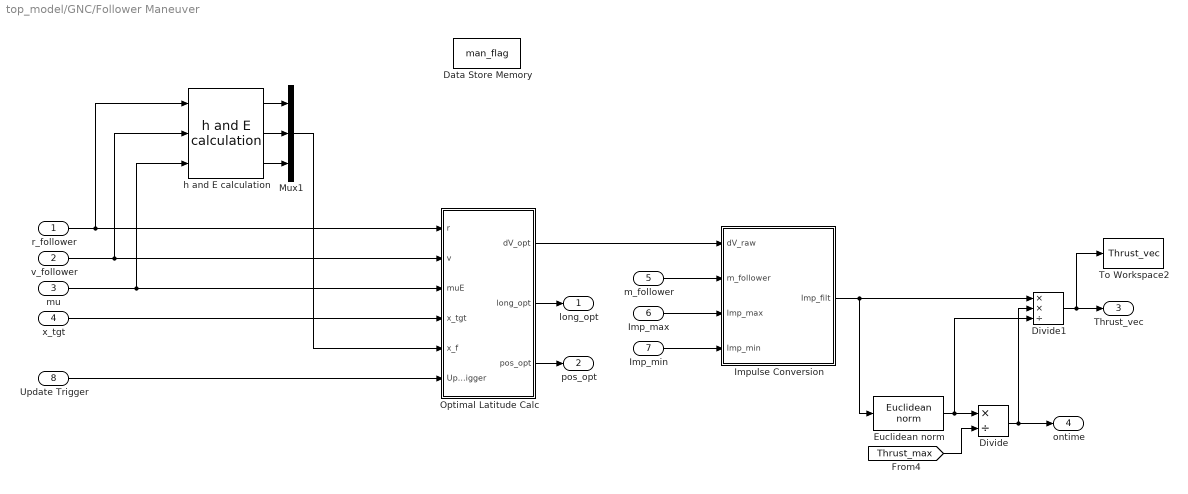
== system top_model/GNC/Follower Maneuver ==
  r_follower : Inport
  v_follower : Inport  Port=2
  mu : Inport  Port=3
  x_tgt : Inport  Port=4
  m_follower : Inport  Port=5
  Imp_max : Inport  Port=6
  Imp_min : Inport  Port=7
  Update Trigger : Inport  Port=8
  Data Store Memory : DataStoreMemory  DataStoreName=man_flag  WriteAfterWriteMsg=warning  WriteAfterReadMsg=warning  ShowAdditionalParam=off
  Divide : Product  Inputs=*/
  Divide1 : Product  Inputs=**/
  Euclidean norm : hEemethod/Math Operations/Euclidean norm
      settings: SourceProductName=HEe Method Library
  Impulse Conversion : MATLAB Function  TreatAsAtomicUnit=on
  Mux1 : Mux  Inputs=3
  Optimal Latitude Calc : Subsystem
  To Workspace2 : ToWorkspace  VariableName=Thrust_vec  SaveFormat=Timeseries  SampleTime=-1
  h and E calculation : hEemethod/Math Operations/h and E calculation
      settings: SourceProductName=HEe Method Library
  long_opt : Outport
  pos_opt : Outport  Port=2
  Thrust_vec : Outport  Port=3
  ontime : Outport  Port=4
  wires:
  r_follower/1 -> h and E calculation/1, Optimal Latitude Calc/1("r ")
  h and E calculation/1 -> Mux1/1
  h and E calculation/2 -> Mux1/2
  Mux1/1 -> Optimal Latitude Calc/5(x_f)
  x_tgt/1 -> Optimal Latitude Calc/4(x_tgt)
  mu/1 -> h and E calculation/3, Optimal Latitude Calc/3(muE)
  v_follower/1 -> h and E calculation/2, Optimal Latitude Calc/2("v ")
  h and E calculation/3 -> Mux1/3
  Optimal Latitude Calc/2(long_opt) -> long_opt/1
  Optimal Latitude Calc/1(dV_opt) -> Impulse Conversion/1(dV_raw)
  Imp_min/1 -> Impulse Conversion/4(Imp_min)
  Imp_max/1 -> Impulse Conversion/3(Imp_max)
  m_follower/1 -> Impulse Conversion/2(m_follower)
  Update Trigger/1 -> Optimal Latitude Calc/6(Update Trigger)
  Optimal Latitude Calc/3(pos_opt) -> pos_opt/1
  Euclidean norm/1 -> Divide1/3, Divide/1
  Divide1/1 -> To Workspace2/1, Thrust_vec/1
  [Thrust_max] -> Divide/2
  Divide/1 -> Divide1/2, ontime/1
  Impulse Conversion/1(Imp_filt) -> Euclidean norm/1, Divide1/1

== system top_model/GNC/Follower Orbital Elements ==
  r : Inport
  v : Inport  Port=2
  Follower True Anomaly : hEemethod/Math Operations/True Anomaly
      settings: SourceProductName=HEe Method Library
  Mux : Mux  Inputs=3
  Orbital Elements : hEemethod/Math Operations/Orbital Elements
      settings: SourceProductName=HEe Method Library
  h and E calculation : hEemethod/Math Operations/h and E calculation
      settings: SourceProductName=HEe Method Library
  a : Outport
  e : Outport  Port=2
  i : Outport  Port=3
  Ω : Outport  Port=4
  ω : Outport  Port=5
  θ : Outport  Port=6
  wires:
  h and E calculation/1 -> Mux/1
  Orbital Elements/5 -> ω/1
  Orbital Elements/2 -> e/1
  Orbital Elements/3 -> i/1
  Orbital Elements/1 -> a/1
  r/1 -> Follower True Anomaly/1, h and E calculation/1
  Orbital Elements/4 -> Ω/1
  v/1 -> Follower True Anomaly/2, h and E calculation/2
  Mux/1 -> Orbital Elements/1
  h and E calculation/2 -> Mux/2
  h and E calculation/3 -> Mux/3
  [muE] -> Follower True Anomaly/3, Orbital Elements/2, h and E calculation/3
  Follower True Anomaly/1 -> θ/1

== system top_model/GNC/Leader Orbital Elements ==
  r : Inport
  v : Inport  Port=2
  Follower True Anomaly : hEemethod/Math Operations/True Anomaly
      settings: SourceProductName=HEe Method Library
  Mux : Mux  Inputs=3
  Orbital Elements : hEemethod/Math Operations/Orbital Elements
      settings: SourceProductName=HEe Method Library
  h and E calculation : hEemethod/Math Operations/h and E calculation
      settings: SourceProductName=HEe Method Library
  a : Outport
  e : Outport  Port=2
  i : Outport  Port=3
  Ω : Outport  Port=4
  ω : Outport  Port=5
  θ : Outport  Port=6
  wires:
  h and E calculation/1 -> Mux/1
  Orbital Elements/5 -> ω/1
  Orbital Elements/2 -> e/1
  Orbital Elements/3 -> i/1
  Orbital Elements/1 -> a/1
  r/1 -> Follower True Anomaly/1, h and E calculation/1
  Orbital Elements/4 -> Ω/1
  v/1 -> Follower True Anomaly/2, h and E calculation/2
  Mux/1 -> Orbital Elements/1
  h and E calculation/2 -> Mux/2
  h and E calculation/3 -> Mux/3
  [muE] -> Follower True Anomaly/3, Orbital Elements/2, h and E calculation/3
  Follower True Anomaly/1 -> θ/1

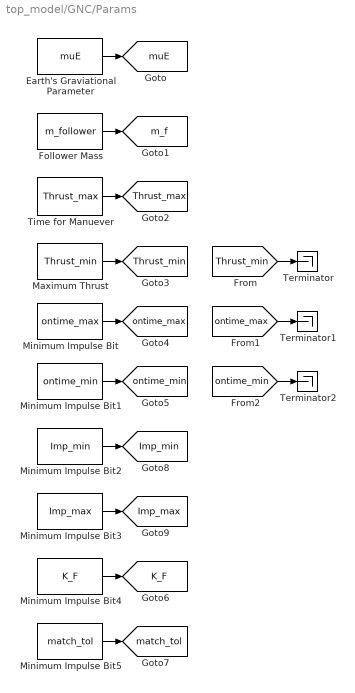
== system top_model/GNC/Params ==
  Earth's Graviational Parameter : Constant  Value=muE
  Follower Mass : Constant  Value=m_follower
  Maximum Thrust : Constant  Value=Thrust_min
  Minimum Impulse Bit : Constant  Value=ontime_max
  Minimum Impulse Bit1 : Constant  Value=ontime_min
  Minimum Impulse Bit2 : Constant  Value=Imp_min
  Minimum Impulse Bit3 : Constant  Value=Imp_max
  Minimum Impulse Bit4 : Constant  Value=K_F
  Minimum Impulse Bit5 : Constant  Value=match_tol
  Terminator : Terminator
  Terminator1 : Terminator
  Terminator2 : Terminator
  Time for Manuever : Constant  Value=Thrust_max
  tag scope: Imp_max=global, Imp_min=global, K_F=global, Thrust_max=global, Thrust_min=global, m_f=global, match_tol=global, muE=global, ontime_max=global, ontime_min=global
  wires:
  Time for Manuever/1 -> [Thrust_max]
  Follower Mass/1 -> [m_f]
  Earth's Graviational Parameter/1 -> [muE]
  Maximum Thrust/1 -> [Thrust_min]
  Minimum Impulse Bit/1 -> [ontime_max]
  Minimum Impulse Bit1/1 -> [ontime_min]
  Minimum Impulse Bit2/1 -> [Imp_min]
  Minimum Impulse Bit3/1 -> [Imp_max]
  [Thrust_min] -> Terminator/1
  [ontime_max] -> Terminator1/1
  [ontime_min] -> Terminator2/1
  Minimum Impulse Bit4/1 -> [K_F]
  Minimum Impulse Bit5/1 -> [match_tol]

== system top_model/LDR_Plant/Cross ==
  A : Inport
  B : Inport  Port=2
  Mux4 : Mux  Inputs=3
  Product{,1..5} (6 alike) : Product  SaturateOnIntegerOverflow=on  InputSameDT=on  OutDataTypeStr=Inherit: Same as first input
  Sum : Sum  Inputs=+-  SaturateOnIntegerOverflow=on  InputSameDT=on  OutDataTypeStr=Inherit: Same as first input
  Sum1 : Sum  Inputs=+-  SaturateOnIntegerOverflow=on  InputSameDT=on  OutDataTypeStr=Inherit: Same as first input
  Sum2 : Sum  Inputs=+-  SaturateOnIntegerOverflow=on  InputSameDT=on  OutDataTypeStr=Inherit: Same as first input
  demux2 : Demux  Outputs=3
  demux3 : Demux  Outputs=3
  AxB : Outport  InitialOutput=0
  wires:
  Mux4/1 -> AxB/1
  Sum2/1 -> Mux4/3
  Sum1/1 -> Mux4/2
  Sum/1 -> Mux4/1
  Product5/1 -> Sum2/2
  Product4/1 -> Sum2/1
  Product3/1 -> Sum1/2
  Product2/1 -> Sum1/1
  Product1/1 -> Sum/2
  Product/1 -> Sum/1
  demux3/1 -> Product5/2, Product2/2
  demux2/2 -> Product5/1, Product/1
  demux3/2 -> Product4/2, Product1/2
  demux2/1 -> Product4/1, Product3/1
  demux3/3 -> Product3/2, Product/2
  demux2/3 -> Product2/1, Product1/1
  B/1 -> demux3/1
  A/1 -> demux2/1
